simulink model "pid1"  (R2023b)
settings: Solver=VariableStepAuto  StartTime=0.0  StopTime=10.0  RelTol=1e-3
libraries: simulink x1
settings Model: Creator=21917  LastModifiedBy=21917

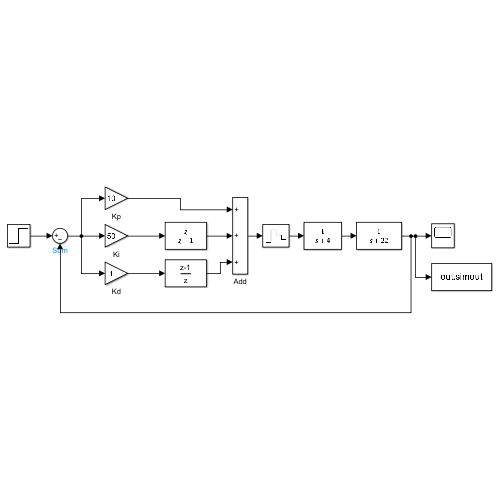
[thumbnail: Simulink's stored preview of the top-level diagram]
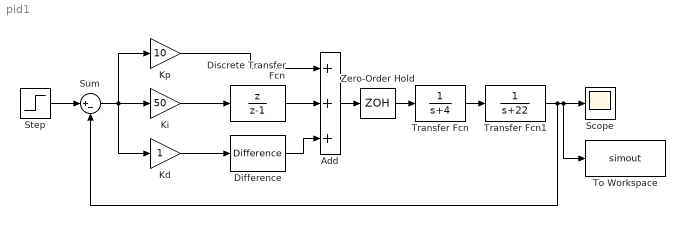
== system pid1 ==
  Add : Sum  Inputs=+++
  Difference : simulink/Discrete/Difference  ICPrevInput=0.0  OutMin=[]  OutMax=[]  OutDataType=fixdt(1, 16)  OutScaling=2^-10  DoSatur=off
  Discrete Transfer Fcn : DiscreteTransferFcn  Numerator=[1 0]  Denominator=[1 -1]
  Kd : Gain
  Ki : Gain  Gain=50
  Kp : Gain  Gain=10
  Scope : Scope
  Step : Step  SampleTime=0
  Sum : Sum  Inputs=|+-
  To Workspace : ToWorkspace  VariableName=simout  SaveFormat=Timeseries  SampleTime=-1
  Transfer Fcn : TransferFcn  Denominator=[1 4]
  Transfer Fcn1 : TransferFcn  Denominator=[1 22]
  Zero-Order Hold : ZeroOrderHold  SampleTime=-1
  wires:
  Step/1 -> Sum/1
  Sum/1 -> Kd/1, Ki/1, Kp/1
  Kd/1 -> Difference/1
  Ki/1 -> Discrete Transfer Fcn/1
  Discrete Transfer Fcn/1 -> Add/2
  Difference/1 -> Add/3
  Kp/1 -> Add/1
  Add/1 -> Zero-Order Hold/1
  Zero-Order Hold/1 -> Transfer Fcn/1
  Transfer Fcn/1 -> Transfer Fcn1/1
  Transfer Fcn1/1 -> Sum/2, Scope/1, To Workspace/1
